simulink model "improved_DTC_model"  (R2024b)
settings: Solver=ode23tb  StartTime=0.0  StopTime=0.4  RelTol=1e-3
InitFcn:
  | pn = 4;
  | Ld = 8.5e-3;
  | Lq = 8.5e-3;
  | R = 1.2;
  | phi = 0.175;
  | J = 0.0008;
  | B = 0.000;
values from neighbouring files (symbols this model uses):
  N = 4*a + 2*b + c    (= 7)    [sector.m]
libraries: spsGroundLib x1, spsUniversalBridgeLib x1, spsPermanentMagnetSynchronousMachineLib x1, spsSVPWMGenerator2LevelLib x1, spsThreePhaseVIMeasurementLib x1, spsDCVoltageSourceLib x1, sps_lib x1

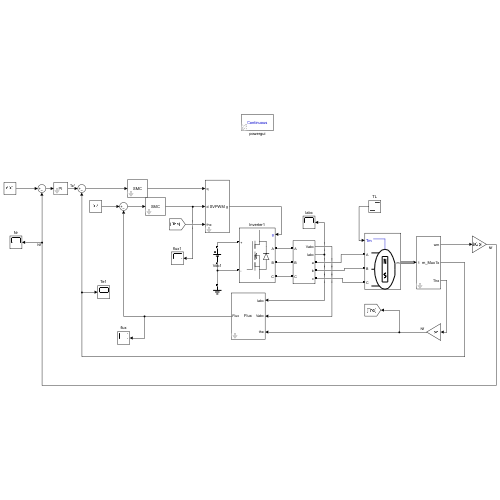
[thumbnail: Simulink's stored preview of the top-level diagram]
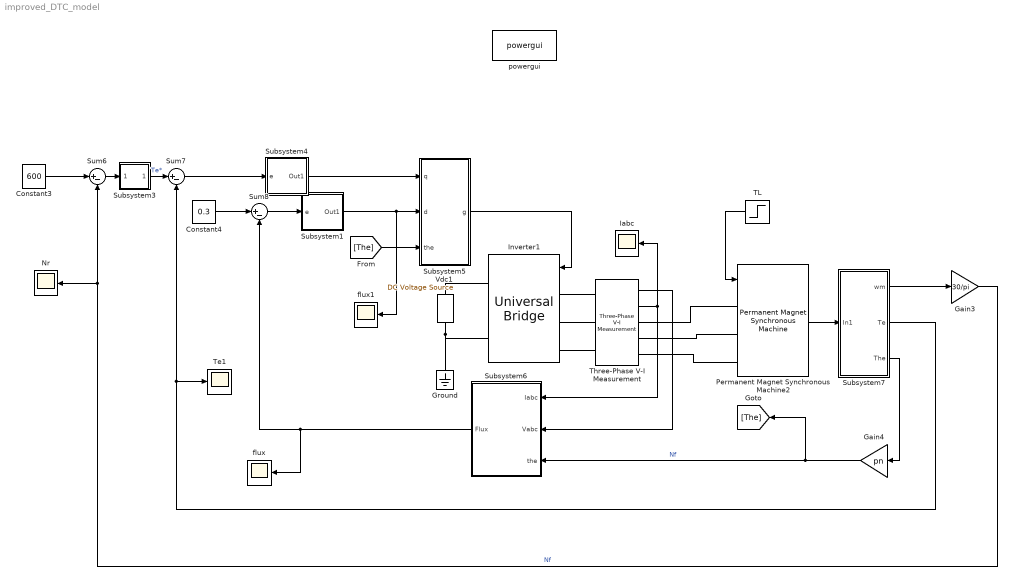
== system improved_DTC_model ==
  Constant3 : Constant  Value=600
  Constant4 : Constant  Value=0.3
  Gain3 : Gain  Gain=30/pi
  Gain4 : Gain  Gain=pn
  Ground : spsGroundLib/Ground  LConnTagsString=a
  Iabc : Scope
  Inverter1 : spsUniversalBridgeLib/Universal Bridge  Arms=3  SnubberResistance=1e5  SnubberCapacitance=inf  Device=MOSFET / Diodes  Ron=1e-3  Lon=0  ForwardVoltages="[  0  0  ]"  ForwardVoltage=0  GTOparameters=[ 10e-6 , 20e-6 ]  IGBTparameters=[ 1e-6 , 2e-6 ]  Measurements=None  Measurements_2=None  converterType=Rectifier
  Nr : Scope
  Permanent Magnet Synchronous Machine2 : spsPermanentMagnetSynchronousMachineLib/Permanent Magnet Synchronous Machine  NbPhases=3  FluxDistribution=Sinusoidal  RotorType=Salient-pole  MechanicalLoad=Torque Tm  PresetModel=No  ShowDetailedParameters=on  MeasurementBus=off  Resistance=R  Inductance=8.5e-3  dqInductances=[Ld Lq]  La=0.000395  MachineConstant=Torque Constant (N.m / A_peak)  Flux=0.175  VoltageCst=126.966  TorqueCst=1.05  Flat=120  Mechanical=[J B pn 0]  PolePairs=2  InitialConditions=[0,0, 0,0]  InitialConditions5ph=[0 0 0 0 0 0]  RefAngle=Aligned with phase A axis (original Park)  IterativeDiscreteModel=Trapezoidal non iterative  TsBlock=-1  TsPowergui=0
  Subsystem1 : Subsystem  mask{Kp=100, Ki=5}
      mask prompts: Kp "Kp : Propotional"; Ki "Ki : Integral"
  Subsystem3 : Subsystem
  Subsystem4 : Subsystem  mask{Kp=25, Ki=0.1}
      mask prompts: Kp "Kp : Propotional"; Ki "Ki : Integral"
  Subsystem5 : Subsystem  mask{Vdc=311}
  Subsystem6 : Subsystem
  Subsystem7 : Subsystem
  Sum6 : Sum  Inputs=|+-
  Sum7 : Sum  Inputs=|+-
  Sum8 : Sum  Inputs=|+-
  TL : Step  Time=0.2  After=1.5  SampleTime=0
  Te1 : Scope
  Three-Phase V-I Measurement : spsThreePhaseVIMeasurementLib/Three-Phase V-I Measurement  VoltageMeasurement=phase-to-ground  SetLabelV=off  LabelV=Vabc  Vpu=off  VpuLL=off  CurrentMeasurement=yes  SetLabelI=off  LabelI=Iabc  Ipu=off  Pbase=100e6  Vbase=500e3  OutputType=Complex  PhasorSimulation=off  PSBequivalent=0
  Vdc1 : spsDCVoltageSourceLib/DC Voltage Source  Amplitude=311  Measurements=None
  flux : Scope
  flux1 : Scope
  powergui : sps_lib/powergui  Priority=1  SimulationMode=Continuous  SampleTime=10e-6  frequency=60  Iterations=50  frequencyindice=0  Pbase=100e6  ErrMax=1e-4  UnitsV=kV  UnitsW=MW  buscounter=0  FunctionMessages=off  echomessages=off  EnableUseOfTLC=off  CurrentSourceSwitches=off  DisableSnubberDevices=off  DisableRonSwitches=off  DisableVfSwitches=off  DisplayEquations=off  AutomaticDiscreteSolvers=off  SolverType=Tustin/Backward Euler (TBE)  Interpol=off  ExternalGateDelay=off  methode=off  Ts=100  x0status=blocks  SPID=on  SwTol=0  HookPort=off  NonlinearTolerance=1e-4  nMaxIteration=100  ContinueOnMaxIteration=off  RestoreLinks=warning  ResistiveCurrentMeasurement=off  Frange=[0:2:500]  Ylog=off  Xlog=on  ShowGrid=off  save=off  variable=ZData  structure=0  ZoomFFT=off  StartTime=0.0  cycles=1  DisplayStyle=1  fundamental=60  FreqAxis=off  MaxFrequency=1000  frequencyindicesteady=1  RmsSteady=1  display=off
  wires:
  Three-Phase V-I Measurement/2 -> Subsystem6/1(Iabc), Iabc/1
  Sum7/1 -> Subsystem4/1(e)
  Sum6/1 -> Subsystem3/1(Input)
  Three-Phase V-I Measurement/1 -> Subsystem6/2(Vabc)
  Permanent Magnet Synchronous Machine2/1 -> Subsystem7/1(In1)
  Subsystem3/1(output) -> Sum7/1  "Te*"
  TL/1 -> Permanent Magnet Synchronous Machine2/1
  Constant3/1 -> Sum6/1
  Gain3/1 -> Nr/1, Sum6/2  "Nf"
  Subsystem7/2(Te) -> Sum7/2, Te1/1
  Subsystem5/1(g) -> Inverter1/1
  Subsystem7/1(wm) -> Gain3/1
  Gain4/1 -> Subsystem6/3(the), [The]  "Nf"
  Subsystem7/3(The) -> Gain4/1
  Constant4/1 -> Sum8/1
  Subsystem6/1(Flux) -> flux/1, Sum8/2
  [The] -> Subsystem5/3(the)
  Subsystem4/1(Out1) -> Subsystem5/1(q)
  Sum8/1 -> Subsystem1/1(e)
  Subsystem1/1(Out1) -> flux1/1, Subsystem5/2(d)
  connections:
  Vdc1/LConn1 -- Inverter1/RConn2 -- Ground/LConn1
  Three-Phase V-I Measurement/LConn3 -- Inverter1/LConn3
  Permanent Magnet Synchronous Machine2/LConn1 -- Three-Phase V-I Measurement/RConn1
  Vdc1/RConn1 -- Inverter1/RConn1
  Three-Phase V-I Measurement/LConn2 -- Inverter1/LConn2
  Three-Phase V-I Measurement/LConn1 -- Inverter1/LConn1
  Permanent Magnet Synchronous Machine2/LConn3 -- Three-Phase V-I Measurement/RConn3
  Permanent Magnet Synchronous Machine2/LConn2 -- Three-Phase V-I Measurement/RConn2

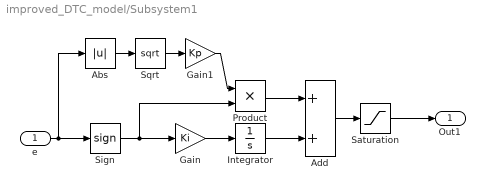
== system improved_DTC_model/Subsystem1 ==
  e : Inport
  Abs : Abs  SaturateOnIntegerOverflow=off
  Add : Sum
  Gain : Gain  Gain=Ki
  Gain1 : Gain  Gain=Kp
  Integrator : Integrator
  Product : Product
  Saturation : Saturate  UpperLimit=100  LowerLimit=-100
  Sign : Signum
  Sqrt : Sqrt
  Out1 : Outport
  wires:
  e/1 -> Abs/1, Sign/1
  Sign/1 -> Product/2, Gain/1
  Gain1/1 -> Product/1
  Gain/1 -> Integrator/1
  Product/1 -> Add/1
  Integrator/1 -> Add/2
  Abs/1 -> Sqrt/1
  Sqrt/1 -> Gain1/1
  Add/1 -> Saturation/1
  Saturation/1 -> Out1/1

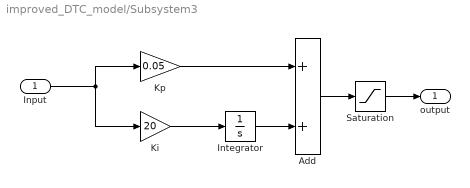
== system improved_DTC_model/Subsystem3 ==
  Input : Inport
  Add : Sum
  Integrator : Integrator
  Ki : Gain  Gain=20
  Kp : Gain  Gain=0.05
  Saturation : Saturate  UpperLimit=50  LowerLimit=-50
  output : Outport
  wires:
  Input/1 -> Ki/1, Kp/1
  Ki/1 -> Integrator/1
  Integrator/1 -> Add/2
  Kp/1 -> Add/1
  Add/1 -> Saturation/1
  Saturation/1 -> output/1

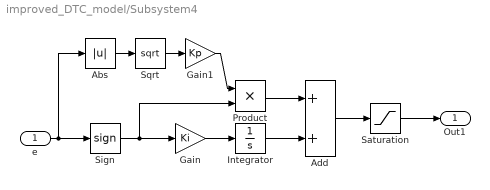
== system improved_DTC_model/Subsystem4 ==
  e : Inport
  Abs : Abs  SaturateOnIntegerOverflow=off
  Add : Sum
  Gain : Gain  Gain=Ki
  Gain1 : Gain  Gain=Kp
  Integrator : Integrator
  Product : Product
  Saturation : Saturate  UpperLimit=150  LowerLimit=-150
  Sign : Signum
  Sqrt : Sqrt
  Out1 : Outport
  wires:
  e/1 -> Abs/1, Sign/1
  Sign/1 -> Product/2, Gain/1
  Gain1/1 -> Product/1
  Gain/1 -> Integrator/1
  Product/1 -> Add/1
  Integrator/1 -> Add/2
  Abs/1 -> Sqrt/1
  Sqrt/1 -> Gain1/1
  Add/1 -> Saturation/1
  Saturation/1 -> Out1/1

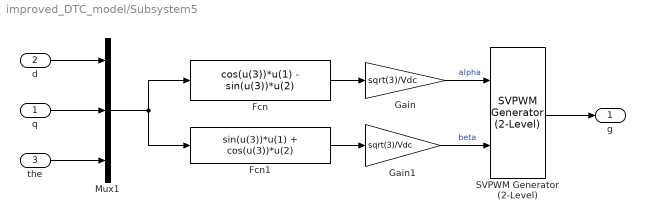
== system improved_DTC_model/Subsystem5 ==
  q : Inport
  d : Inport  Port=2
  the : Inport  Port=3
  Fcn : Fcn  Expr=cos(u(3))*u(1) - sin(u(3))*u(2)
  Fcn1 : Fcn  Expr=sin(u(3))*u(1) + cos(u(3))*u(2)
  Gain : Gain  Gain=sqrt(3)/Vdc
  Gain1 : Gain  Gain=sqrt(3)/Vdc
  Mux1 : Mux  Inputs=3
  SVPWM Generator (2-Level) : spsSVPWMGenerator2LevelLib/SVPWM Generator (2-Level)  InputType=alpha-beta components  SwitchingPattern=Pattern #1  Fc=10e3  ParUref=[0.8 -30 50]  Ts=0
  g : Outport
  wires:
  q/1 -> Mux1/2
  Fcn/1 -> Gain/1
  d/1 -> Mux1/1
  Fcn1/1 -> Gain1/1
  SVPWM Generator (2-Level)/1 -> g/1
  Mux1/1 -> Fcn/1, Fcn1/1
  the/1 -> Mux1/3
  Gain/1 -> SVPWM Generator (2-Level)/1  "alpha"
  Gain1/1 -> SVPWM Generator (2-Level)/2  "beta"

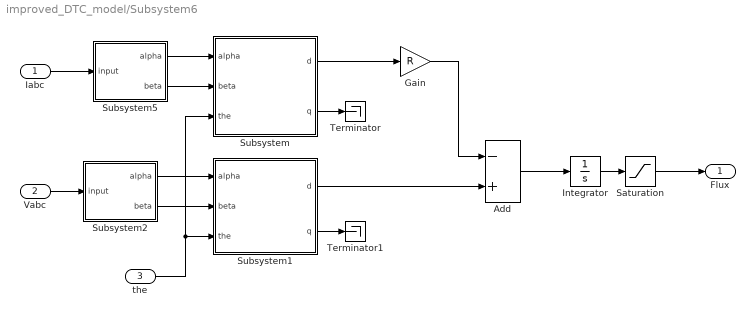
== system improved_DTC_model/Subsystem6 ==
  Iabc : Inport
  Vabc : Inport  Port=2
  the : Inport  Port=3
  Add : Sum  Inputs=-+
  Gain : Gain  Gain=R
  Integrator : Integrator
  Saturation : Saturate  UpperLimit=0.35  LowerLimit=-0.35
  Subsystem : Subsystem
  Subsystem1 : Subsystem
  Subsystem2 : Subsystem
  Subsystem5 : Subsystem
  Terminator : Terminator
  Terminator1 : Terminator
  Flux : Outport
  wires:
  Subsystem5/1(alpha) -> Subsystem/1(alpha)
  Subsystem5/2(beta) -> Subsystem/2(beta)
  Subsystem2/2(beta) -> Subsystem1/2(beta)
  Subsystem2/1(alpha) -> Subsystem1/1(alpha)
  Iabc/1 -> Subsystem5/1(input)
  Vabc/1 -> Subsystem2/1(input)
  the/1 -> Subsystem/3(the), Subsystem1/3(the)
  Subsystem/2(q) -> Terminator/1
  Subsystem1/2(q) -> Terminator1/1
  Subsystem/1(d) -> Gain/1
  Subsystem1/1(d) -> Add/2
  Gain/1 -> Add/1
  Add/1 -> Integrator/1
  Integrator/1 -> Saturation/1
  Saturation/1 -> Flux/1

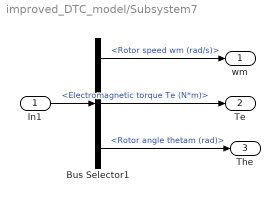
== system improved_DTC_model/Subsystem7 ==
  In1 : Inport
  Bus Selector1 : BusSelector  OutputSignals=Rotor speed wm (rad/s),Electromagnetic torque Te (N*m),Rotor angle thetam (rad)
  wm : Outport
  Te : Outport  Port=2
  The : Outport  Port=3
  wires:
  In1/1 -> Bus Selector1/1
  Bus Selector1/1 -> wm/1  "<Rotor speed wm (rad/s)>"
  Bus Selector1/2 -> Te/1  "<Electromagnetic torque Te (N*m)>"
  Bus Selector1/3 -> The/1  "<Rotor angle thetam (rad)>"

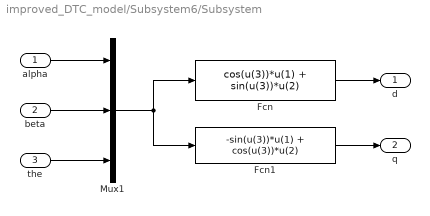
== system improved_DTC_model/Subsystem6/Subsystem ==
  alpha : Inport
  beta : Inport  Port=2
  the : Inport  Port=3
  Fcn : Fcn  Expr=cos(u(3))*u(1) + sin(u(3))*u(2)
  Fcn1 : Fcn  Expr=-sin(u(3))*u(1) + cos(u(3))*u(2)
  Mux1 : Mux  Inputs=3
  d : Outport
  q : Outport  Port=2
  wires:
  Fcn/1 -> d/1
  Mux1/1 -> Fcn/1, Fcn1/1
  the/1 -> Mux1/3
  beta/1 -> Mux1/2
  Fcn1/1 -> q/1
  alpha/1 -> Mux1/1

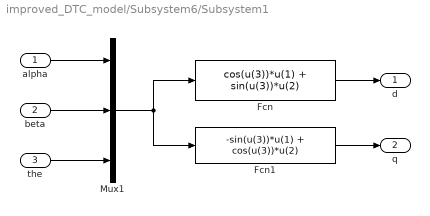
== system improved_DTC_model/Subsystem6/Subsystem1 ==
  alpha : Inport
  beta : Inport  Port=2
  the : Inport  Port=3
  Fcn : Fcn  Expr=cos(u(3))*u(1) + sin(u(3))*u(2)
  Fcn1 : Fcn  Expr=-sin(u(3))*u(1) + cos(u(3))*u(2)
  Mux1 : Mux  Inputs=3
  d : Outport
  q : Outport  Port=2
  wires:
  Fcn/1 -> d/1
  Mux1/1 -> Fcn/1, Fcn1/1
  the/1 -> Mux1/3
  beta/1 -> Mux1/2
  Fcn1/1 -> q/1
  alpha/1 -> Mux1/1

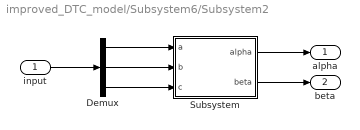
== system improved_DTC_model/Subsystem6/Subsystem2 ==
  input : Inport
  Demux : Demux  Outputs=3
  Subsystem : Subsystem
  alpha : Outport
  beta : Outport  Port=2
  wires:
  input/1 -> Demux/1
  Demux/1 -> Subsystem/1(a)
  Demux/2 -> Subsystem/2(b)
  Demux/3 -> Subsystem/3(c)
  Subsystem/1(alpha) -> alpha/1
  Subsystem/2(beta) -> beta/1

== system improved_DTC_model/Subsystem6/Subsystem5 ==
  input : Inport
  Demux : Demux  Outputs=3
  Subsystem : Subsystem
  alpha : Outport
  beta : Outport  Port=2
  wires:
  input/1 -> Demux/1
  Demux/1 -> Subsystem/1(a)
  Demux/2 -> Subsystem/2(b)
  Demux/3 -> Subsystem/3(c)
  Subsystem/1(alpha) -> alpha/1
  Subsystem/2(beta) -> beta/1

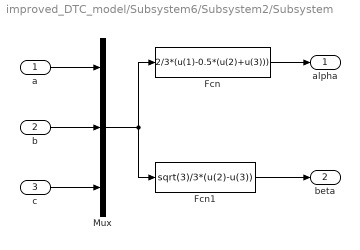
== system improved_DTC_model/Subsystem6/Subsystem2/Subsystem ==
  a : Inport
  b : Inport  Port=2
  c : Inport  Port=3
  Fcn : Fcn  Expr=2/3*(u(1)-0.5*(u(2)+u(3)))
  Fcn1 : Fcn  Expr=sqrt(3)/3*(u(2)-u(3))
  Mux : Mux  Inputs=3
  alpha : Outport
  beta : Outport  Port=2
  wires:
  a/1 -> Mux/1
  b/1 -> Mux/2
  c/1 -> Mux/3
  Mux/1 -> Fcn/1, Fcn1/1
  Fcn/1 -> alpha/1
  Fcn1/1 -> beta/1

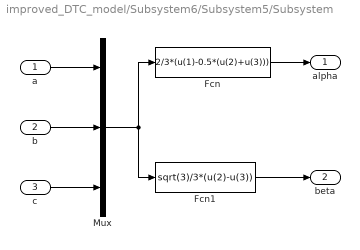
== system improved_DTC_model/Subsystem6/Subsystem5/Subsystem ==
  a : Inport
  b : Inport  Port=2
  c : Inport  Port=3
  Fcn : Fcn  Expr=2/3*(u(1)-0.5*(u(2)+u(3)))
  Fcn1 : Fcn  Expr=sqrt(3)/3*(u(2)-u(3))
  Mux : Mux  Inputs=3
  alpha : Outport
  beta : Outport  Port=2
  wires:
  a/1 -> Mux/1
  b/1 -> Mux/2
  c/1 -> Mux/3
  Mux/1 -> Fcn/1, Fcn1/1
  Fcn/1 -> alpha/1
  Fcn1/1 -> beta/1
